simulink model "vehicle_powertrain_model"  (R2019b)
settings: Solver=VariableStepAuto  StartTime=0.0  StopTime=10.0  RelTol=1e-3
settings Model: Creator=karth  LastModifiedBy=karth

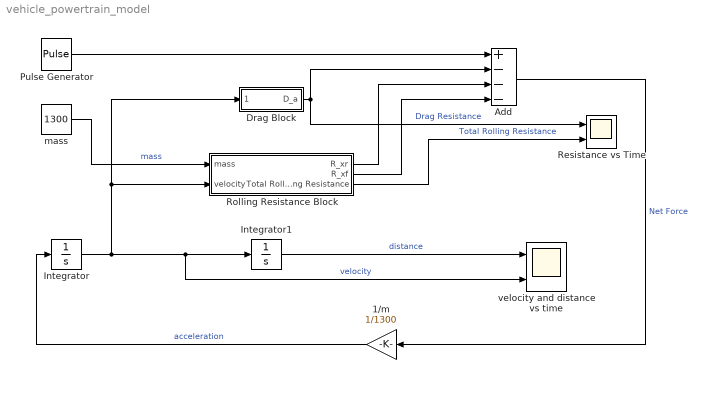
== system vehicle_powertrain_model ==
  1/m : Gain  Gain=1/1300
  Add : Sum  Inputs=+---
  Drag Block : Subsystem
  Integrator : Integrator
  Integrator1 : Integrator
  Pulse Generator : DiscretePulseGenerator  PulseType=Time based  Amplitude=1500  PulseWidth=30
  Resistance vs Time : Scope  NumInputPorts=2
  Rolling Resistance Block : Subsystem
  mass : Constant  Value=1300
  velocity and distance vs time : Scope  NumInputPorts=2
  wires:
  1/m/1 -> Integrator/1  "acceleration"
  Integrator/1 -> Drag Block/1(velocity), Rolling Resistance Block/2(velocity), velocity and distance vs time/2, Integrator1/1  "velocity"
  Integrator1/1 -> velocity and distance vs time/1  "distance"
  mass/1 -> Rolling Resistance Block/1(mass)  "mass"
  Drag Block/1(D_a) -> Add/2, Resistance vs Time/1  "Drag Resistance"
  Rolling Resistance Block/1(R_xr) -> Add/3
  Rolling Resistance Block/2(R_xf) -> Add/4
  Add/1 -> 1/m/1  "Net Force"
  Rolling Resistance Block/3(Total Rolling Resistance) -> Resistance vs Time/2  "Total Rolling Resistance"
  Pulse Generator/1 -> Add/1

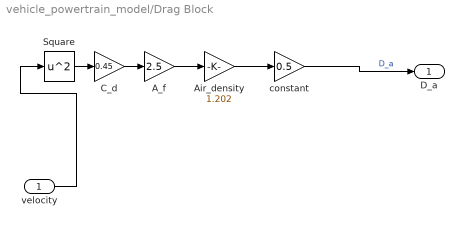
== system vehicle_powertrain_model/Drag Block ==
  velocity : Inport
  A_f : Gain  Gain=2.5
  Air_density : Gain  Gain=1.202
  C_d : Gain  Gain=0.45
  Square : Math  Operator=square  SignedPower=off  SaturateOnIntegerOverflow=on
  constant : Gain  Gain=0.5
  D_a : Outport
  wires:
  Square/1 -> C_d/1
  Air_density/1 -> constant/1
  constant/1 -> D_a/1  "D_a"
  C_d/1 -> A_f/1
  velocity/1 -> Square/1
  A_f/1 -> Air_density/1

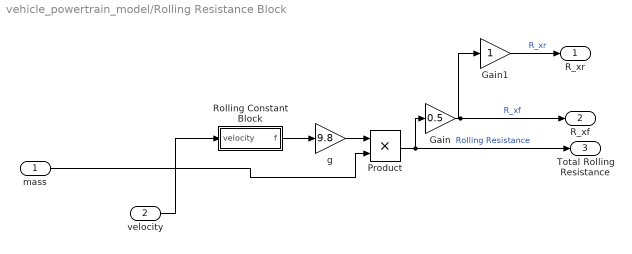
== system vehicle_powertrain_model/Rolling Resistance Block ==
  mass : Inport
  velocity : Inport  Port=2
  Gain : Gain  Gain=0.5
  Gain1 : Gain
  Product : Product
  Rolling Constant Block : Subsystem
  g : Gain  Gain=9.8
  R_xr : Outport
  R_xf : Outport  Port=2
  Total Rolling Resistance : Outport  Port=3
  wires:
  Product/1 -> Total Rolling Resistance/1, Gain/1  "Rolling Resistance"
  Gain/1 -> R_xf/1, Gain1/1  "R_xf"
  velocity/1 -> Rolling Constant Block/1(velocity)
  g/1 -> Product/1
  Rolling Constant Block/1(f) -> g/1
  Gain1/1 -> R_xr/1  "R_xr"
  mass/1 -> Product/2

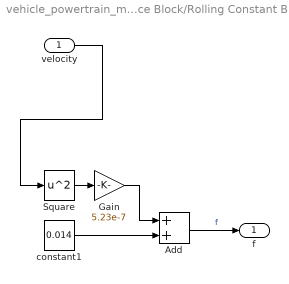
== system vehicle_powertrain_model/Rolling Resistance Block/Rolling Constant Block ==
  velocity : Inport
  Add : Sum
  Gain : Gain  Gain=5.23e-7
  Square : Math  Operator=square  SignedPower=off  SaturateOnIntegerOverflow=on
  constant1 : Constant  Value=0.014
  f : Outport
  wires:
  Gain/1 -> Add/1
  Square/1 -> Gain/1
  constant1/1 -> Add/2
  velocity/1 -> Square/1
  Add/1 -> f/1  "f"
